simulink model "mc"  (R2025b)
settings: Solver=ode45  StartTime=0.0  StopTime=simlength  MaxStep=1e-4  RelTol=1e-4
values from neighbouring files (symbols this model uses):
  A = [0 1 0;      0 -b/m Bm*h/m;      0 -Bm*h/L -R/L]    [init_moving_coil.m]
  Aled = eye(4) + Ale*Ts    [init_moving_coil.m]
  B = [0 0 1/L]'    [init_moving_coil.m]
  Bled = Ble*Ts    [init_moving_coil.m]
  Bm = 1    [init_moving_coil.m]
  C = [1 0 0; 0 0 1]    [init_moving_coil.m]
  Cle = [1 0 0 0; 0 0 1 0]    [init_moving_coil.m]
  E = [0 -1/m 0]'    [init_moving_coil.m]
  h = 200e-3    (= 0.2)    [init_moving_coil.m]
  Ked = (Ke_hat+[0 0 0 1])/([Ad-eye(3) Bd; C(1,:)*Ad C(1,:)*Bd])    [init_moving_coil.m]
  Lled = place(Aled',Cle',poles_so_led)'    [init_moving_coil.m]
  Tc = 1e-5    (= 1e-05)    [init_moving_coil.m]
  Ts = 1/1e3    (= 0.001)    [init_moving_coil.m]
libraries: ee_lib x1
settings Model: Creator=dabagnara  LastModifiedBy=dbagn
settings SolverCC: AlgebraicLoopSolver=TrustRegion
settings DataIOCC: ReturnWorkspaceOutputs=off
settings DebuggingCC: UnconnectedInputMsg=warning  UnconnectedOutputMsg=warning  UnconnectedLineMsg=warning
settings ModelReferenceCC: EnableRefExpFcnMdlSchedulingChecks=on
settings RTWCC: GPUComputeCapability=3.5

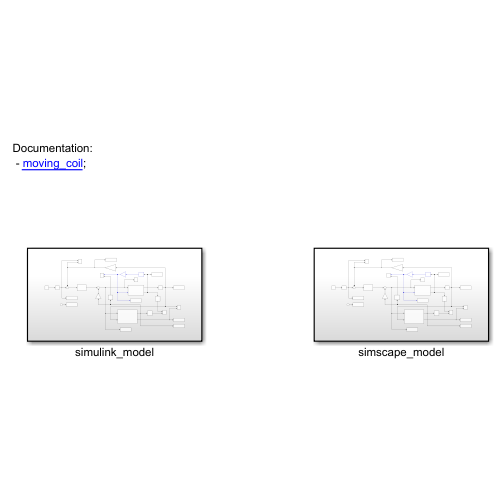
[thumbnail: Simulink's stored preview of the top-level diagram]
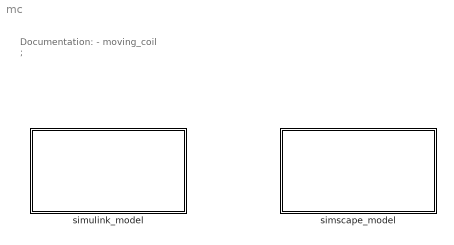
== system mc ==
  note: Documentation:
      | - moving_coil ;
  simscape_model : Subsystem
  simulink_model : Subsystem

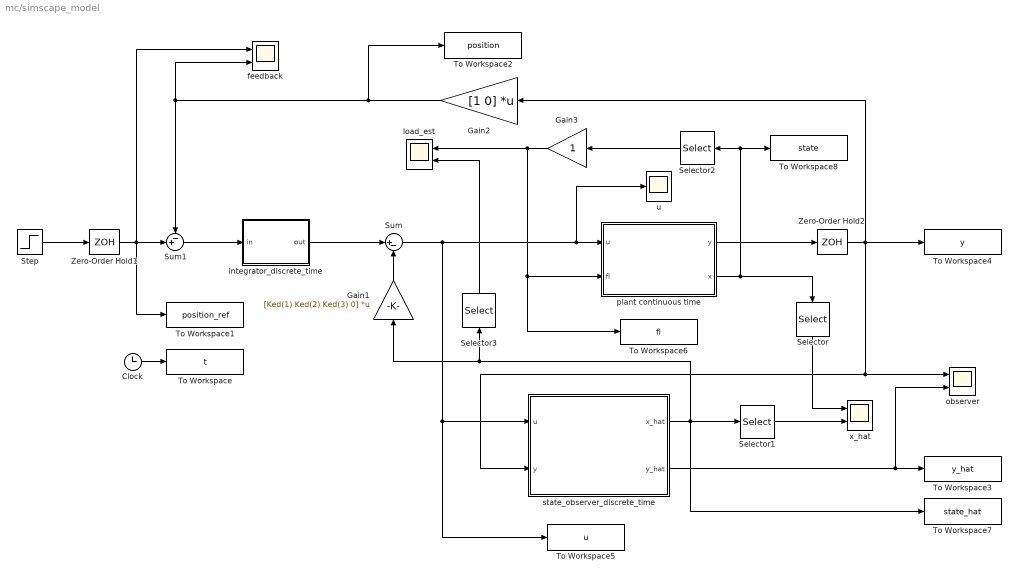
== system mc/simscape_model ==
  Clock : Clock
  Gain1 : Gain  Gain=[Ked(1) Ked(2) Ked(3) 0]  Multiplication=Matrix(K*u)
  Gain2 : Gain  Gain=[1 0]  Multiplication=Matrix(K*u)
  Gain3 : Gain
  Selector : Selector  InputPortWidth=3  IndexOptions=Index vector (dialog)  Indices=2  OutputSizes=1
  Selector1 : Selector  InputPortWidth=4  IndexOptions=Index vector (dialog)  Indices=2  OutputSizes=1
  Selector2 : Selector  InputPortWidth=3  IndexOptions=Index vector (dialog)  Indices=2  OutputSizes=1
  Selector3 : Selector  InputPortWidth=4  IndexOptions=Index vector (dialog)  Indices=4  OutputSizes=1
  Step : Step  Time=0.1  SampleTime=0
  Sum : Sum  Inputs=|+-
  Sum1 : Sum  Inputs=-+|
  To Workspace : ToWorkspace  VariableName=t  SampleTime=Tc
      settings: MaxDataPoints=Nc
  To Workspace1 : ToWorkspace  VariableName=position_ref  SampleTime=Tc
      settings: MaxDataPoints=Nc
  To Workspace2 : ToWorkspace  VariableName=position  SampleTime=Tc
      settings: MaxDataPoints=Nc
  To Workspace3 : ToWorkspace  VariableName=y_hat  SampleTime=Tc
      settings: MaxDataPoints=Nc
  To Workspace4 : ToWorkspace  VariableName=y  SampleTime=Tc
      settings: MaxDataPoints=Nc
  To Workspace5 : ToWorkspace  VariableName=u  SampleTime=Tc
      settings: MaxDataPoints=Nc
  To Workspace6 : ToWorkspace  VariableName=fl  SampleTime=Tc
      settings: MaxDataPoints=Nc
  To Workspace7 : ToWorkspace  VariableName=state_hat  SampleTime=Tc
      settings: MaxDataPoints=Nc
  To Workspace8 : ToWorkspace  VariableName=state  SampleTime=Tc
      settings: MaxDataPoints=Nc
  Zero-Order Hold1 : ZeroOrderHold  SampleTime=Ts
  Zero-Order Hold2 : ZeroOrderHold  SampleTime=Ts
  feedback : Scope  NumInputPorts=2
      settings: ActiveDisplayYMinimum=-0.125  ActiveDisplayYMaximum=1.125
  integrator_discrete_time : Subsystem
  load_est : Scope  NumInputPorts=2
      settings: ActiveDisplayYMinimum=-2.8529  ActiveDisplayYMaximum=14.58894
  observer : Scope  NumInputPorts=2
      settings: ActiveDisplayYMinimum=-11.870884279558481  ActiveDisplayYMaximum=68.425236612925119
  plant continuous time : Subsystem
  state_observer_discrete_time : Subsystem
  u : Scope
      settings: ActiveDisplayYMinimum=-2.39676  ActiveDisplayYMaximum=8.18256  DataLoggingVariableName=ScopeData2
  x_hat : Scope  NumInputPorts=2
      settings: ActiveDisplayYMinimum=-6.8578  ActiveDisplayYMaximum=10.89096  DataLoggingVariableName=ScopeData3
  wires:
  plant continuous time/1(y) -> Zero-Order Hold2/1
  Sum1/1 -> integrator_discrete_time/1(in)
  integrator_discrete_time/1(out) -> Sum/1
  Selector3/1 -> load_est/2
  Selector2/1 -> Gain3/1
  Gain2/1 -> To Workspace2/1, feedback/2, Sum1/1
  Step/1 -> Zero-Order Hold1/1
  Gain1/1 -> Sum/2
  Sum/1 -> state_observer_discrete_time/1(u), To Workspace5/1, plant continuous time/1(u), u/1
  Selector/1 -> x_hat/1
  state_observer_discrete_time/2(y_hat) -> observer/2, To Workspace3/1
  Clock/1 -> To Workspace/1
  Selector1/1 -> x_hat/2
  state_observer_discrete_time/1(x_hat) -> Gain1/1, Selector3/1, To Workspace7/1, Selector1/1
  Zero-Order Hold2/1 -> Gain2/1, To Workspace4/1, observer/1, state_observer_discrete_time/2(y)
  Zero-Order Hold1/1 -> Sum1/2, feedback/1, To Workspace1/1
  Gain3/1 -> load_est/1, To Workspace6/1, plant continuous time/2(fl)
  plant continuous time/2(x) -> Selector/1, Selector2/1, To Workspace8/1

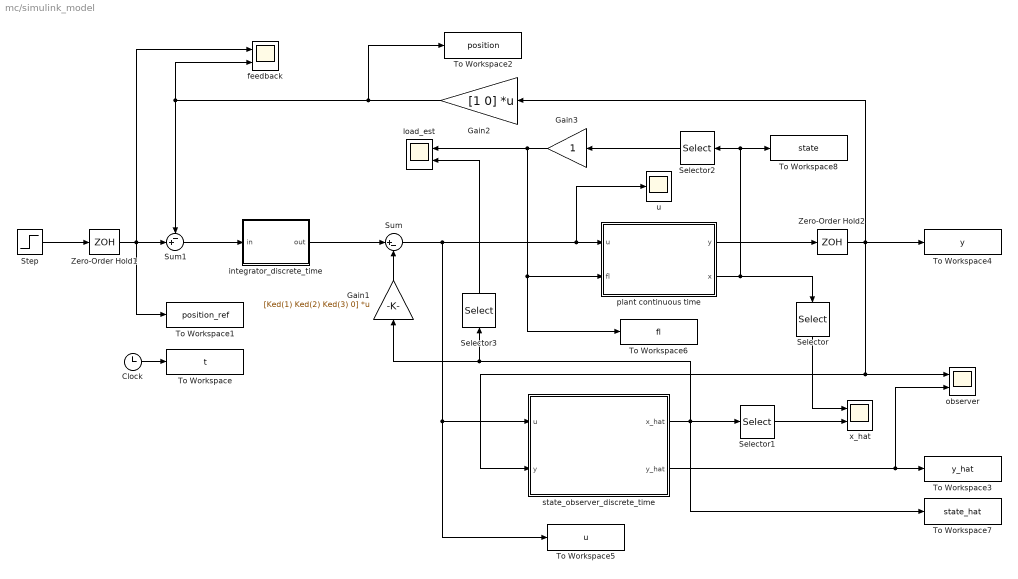
== system mc/simulink_model ==
  Clock : Clock
  Gain1 : Gain  Gain=[Ked(1) Ked(2) Ked(3) 0]  Multiplication=Matrix(K*u)
  Gain2 : Gain  Gain=[1 0]  Multiplication=Matrix(K*u)
  Gain3 : Gain
  Selector : Selector  InputPortWidth=3  IndexOptions=Index vector (dialog)  Indices=2  OutputSizes=1
  Selector1 : Selector  InputPortWidth=4  IndexOptions=Index vector (dialog)  Indices=2  OutputSizes=1
  Selector2 : Selector  InputPortWidth=3  IndexOptions=Index vector (dialog)  Indices=2  OutputSizes=1
  Selector3 : Selector  InputPortWidth=4  IndexOptions=Index vector (dialog)  Indices=4  OutputSizes=1
  Step : Step  Time=0.1  SampleTime=0
  Sum : Sum  Inputs=|+-
  Sum1 : Sum  Inputs=-+|
  To Workspace : ToWorkspace  VariableName=t  SampleTime=Tc
      settings: MaxDataPoints=Nc
  To Workspace1 : ToWorkspace  VariableName=position_ref  SampleTime=Tc
      settings: MaxDataPoints=Nc
  To Workspace2 : ToWorkspace  VariableName=position  SampleTime=Tc
      settings: MaxDataPoints=Nc
  To Workspace3 : ToWorkspace  VariableName=y_hat  SampleTime=Tc
      settings: MaxDataPoints=Nc
  To Workspace4 : ToWorkspace  VariableName=y  SampleTime=Tc
      settings: MaxDataPoints=Nc
  To Workspace5 : ToWorkspace  VariableName=u  SampleTime=Tc
      settings: MaxDataPoints=Nc
  To Workspace6 : ToWorkspace  VariableName=fl  SampleTime=Tc
      settings: MaxDataPoints=Nc
  To Workspace7 : ToWorkspace  VariableName=state_hat  SampleTime=Tc
      settings: MaxDataPoints=Nc
  To Workspace8 : ToWorkspace  VariableName=state  SampleTime=Tc
      settings: MaxDataPoints=Nc
  Zero-Order Hold1 : ZeroOrderHold  SampleTime=Ts
  Zero-Order Hold2 : ZeroOrderHold  SampleTime=Ts
  feedback : Scope  NumInputPorts=2
      settings: ActiveDisplayYMinimum=-0.125  ActiveDisplayYMaximum=1.125
  integrator_discrete_time : Subsystem
  load_est : Scope  NumInputPorts=2
      settings: ActiveDisplayYMinimum=-2.8529  ActiveDisplayYMaximum=14.58894
  observer : Scope  NumInputPorts=2
      settings: ActiveDisplayYMinimum=-11.870884279558481  ActiveDisplayYMaximum=68.425236612925119
  plant continuous time : Subsystem
  state_observer_discrete_time : Subsystem
  u : Scope
      settings: ActiveDisplayYMinimum=-2.39676  ActiveDisplayYMaximum=8.18256  DataLoggingVariableName=ScopeData2
  x_hat : Scope  NumInputPorts=2
      settings: ActiveDisplayYMinimum=-6.8578  ActiveDisplayYMaximum=10.89096  DataLoggingVariableName=ScopeData3
  wires:
  plant continuous time/2(x) -> To Workspace8/1, Selector2/1, Selector/1
  Gain3/1 -> plant continuous time/2(fl), To Workspace6/1, load_est/1
  Zero-Order Hold1/1 -> To Workspace1/1, feedback/1, Sum1/2
  Zero-Order Hold2/1 -> state_observer_discrete_time/2(y), observer/1, To Workspace4/1, Gain2/1
  state_observer_discrete_time/1(x_hat) -> Selector1/1, To Workspace7/1, Selector3/1, Gain1/1
  Selector1/1 -> x_hat/2
  Clock/1 -> To Workspace/1
  state_observer_discrete_time/2(y_hat) -> To Workspace3/1, observer/2
  Selector/1 -> x_hat/1
  Sum/1 -> u/1, plant continuous time/1(u), To Workspace5/1, state_observer_discrete_time/1(u)
  Gain1/1 -> Sum/2
  Step/1 -> Zero-Order Hold1/1
  Gain2/1 -> Sum1/1, feedback/2, To Workspace2/1
  Selector2/1 -> Gain3/1
  Selector3/1 -> load_est/2
  integrator_discrete_time/1(out) -> Sum/1
  Sum1/1 -> integrator_discrete_time/1(in)
  plant continuous time/1(y) -> Zero-Order Hold2/1

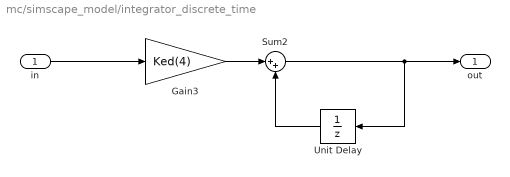
== system mc/simscape_model/integrator_discrete_time ==
  in : Inport
  Gain3 : Gain  Gain=Ked(4)
  Sum2 : Sum  Inputs=|++
  Unit Delay : UnitDelay  SampleTime=Ts  HasFrameUpgradeWarning=on
  out : Outport
  wires:
  Unit Delay/1 -> Sum2/2
  Gain3/1 -> Sum2/1
  in/1 -> Gain3/1
  Sum2/1 -> Unit Delay/1, out/1

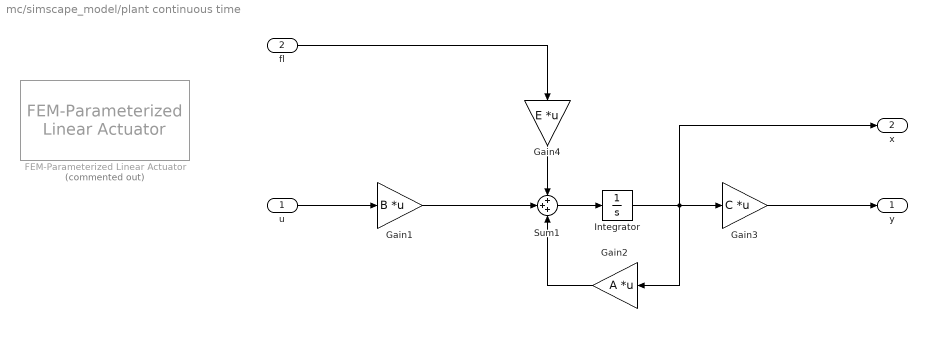
== system mc/simscape_model/plant continuous time ==
  u : Inport
  fl : Inport  Port=2
  FEM-Parameterized Linear Actuator : ee_lib/Electromechanical/Mechatronic Actuators/FEM-Parameterized Linear Actuator  Commented=on  src_type=ee.enum.electromech.femLinearActuator.sourceType.current  iVec=[0, 1] A  xVec=[0, .05, .1, .15, .2] mm  dfluxdiMatrix=L Wb/A  dfluxdxMatrix=Bm*h Wb/m  FluxMatrix=[0, 0, 0, 0, 0; .0085, .0079, .0075, .0071, .0067; .0171, .016, .0151, .0143, .0137; .0254, .0239, .0226, .0215, .0206; .033, .0312, .0297, .0283, .0271; .0396, .0377, .036, .0345, .0331; .0452, .0433, .0415, .0399, .0384; .0495, .0478, .0461, .0446, .0431; .0526, .0512, .0498, .0485, .0472; .0545, .0537, .0528, .0519, .0508; .0554, .0553, .0551, .0548, .0542] Wb  calculate_force_matrix=ee.enum.enable.no  ForceMatrix=[0, 0, 0, 0, 0; -.6, -.5, -.4, -.3, -.3; -2.3, -2, -1.7, -1.4, -1.2; -4.9, -4.3, -3.7, -3.2, -2.7; -8.3, -7.3, -6.4, -5.5, -4.7; -12.2, -10.7, -9.4, -8.2, -7.2; -16.2, -14.4, -12.7, -11.3, -10; -20, -17.9, -15.9, -14.3, -12.9; -23.3, -20.9, -18.8, -17.1, -15.7; -25.7, -23.1, -21.1, -19.4, -18.2; -26.5, -24.1, -22.2, -20.9, -20.1] N  cyclic=ee.enum.isCyclic.unique  interp_method=simscape.enum.interpolation.linear  extrap_method=simscape.enum.extrapolation.linear  R1=14 Ohm  Rm=inf Ohm  lam=1 N*s/m  Mass=0.05 kg  Xmin=0 mm  Xmax=0.2 mm  K_endstop=1e8 N/m  D_endstop=1e4 N*s/m  i_specify=off  i_priority=None  i=0 A  i_nominal_specify=off  i_nominal_value=1  i_nominal_unit=A  F_specify=off  F_priority=None  F=0 N  F_nominal_specify=off  F_nominal_value=1  F_nominal_unit=N  x_specify=off  x_priority=High  x=0 mm  x_nominal_specify=off  x_nominal_value=1  x_nominal_unit=mm  vel_specify=off  vel_priority=High  vel=0 mm/s  vel_nominal_specify=off  vel_nominal_value=1  vel_nominal_unit=mm/s  magnetic_force_specify=off  magnetic_force_priority=None  magnetic_force=0 N  magnetic_force_nominal_specify=off  magnetic_force_nominal_value=1  magnetic_force_nominal_unit=N  alpha=3.93e-3 1/K  Tmeas=25 degC  thermal_mass=100 J/K  T_specify=off  T_priority=High  T=300 K  T_nominal_specify=off  T_nominal_value=1  T_nominal_unit=K
      settings: InternalSimscapePortConfiguration="{\"Bottom\":[],\"Left\":[{\"id\":\"p\",\"label\":\"+\",\"type\":\"foundation.electrical.electrical\"},{\"id\":\"R\",\"label\":\"R\",\"type\":\"foundation.mechanical.translational.translational\"}],\"Right\":[{\"id\":\"n\",\"label\":\"-\",\"type\":\"foundation.electrical.electrical\"},{\"id\":\"C\",\"label\":\"C\",\"type\":\"foundation.mechanical.translational.translational\"}],\"Top\":[]}"
  Gain1 : Gain  Gain=B  Multiplication=Matrix(K*u)
  Gain2 : Gain  Gain=A  Multiplication=Matrix(K*u)
  Gain3 : Gain  Gain=C  Multiplication=Matrix(K*u)
  Gain4 : Gain  Gain=E  Multiplication=Matrix(K*u)
  Integrator : Integrator
  Sum1 : Sum  Inputs=+++
  y : Outport
  x : Outport  Port=2
  wires:
  fl/1 -> Gain4/1
  Gain4/1 -> Sum1/1
  Gain1/1 -> Sum1/2
  Gain2/1 -> Sum1/3
  Gain3/1 -> y/1
  Integrator/1 -> Gain3/1, Gain2/1, x/1
  u/1 -> Gain1/1
  Sum1/1 -> Integrator/1

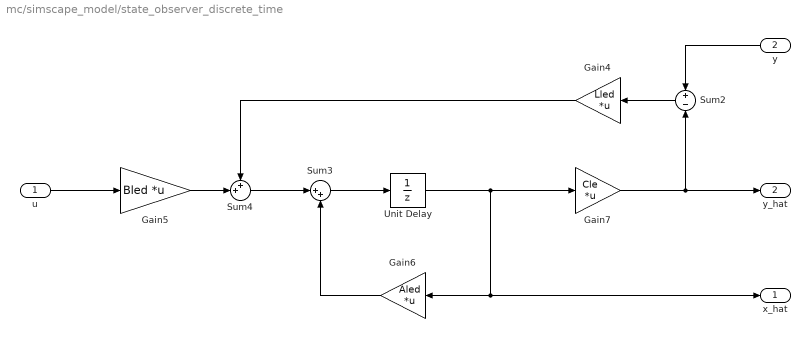
== system mc/simscape_model/state_observer_discrete_time ==
  u : Inport
  y : Inport  Port=2
  Gain4 : Gain  Gain=Lled  Multiplication=Matrix(K*u)
  Gain5 : Gain  Gain=Bled  Multiplication=Matrix(K*u)
  Gain6 : Gain  Gain=Aled  Multiplication=Matrix(K*u)
  Gain7 : Gain  Gain=Cle  Multiplication=Matrix(K*u)
  Sum2 : Sum  Inputs=+-
  Sum3 : Sum  Inputs=|++
  Sum4 : Sum  Inputs=++|
  Unit Delay : UnitDelay  SampleTime=Ts  HasFrameUpgradeWarning=on
  x_hat : Outport
  y_hat : Outport  Port=2
  wires:
  u/1 -> Gain5/1
  Sum4/1 -> Sum3/1
  Gain6/1 -> Sum3/2
  Sum2/1 -> Gain4/1
  Gain5/1 -> Sum4/2
  y/1 -> Sum2/1
  Gain4/1 -> Sum4/1
  Sum3/1 -> Unit Delay/1
  Unit Delay/1 -> x_hat/1, Gain6/1, Gain7/1
  Gain7/1 -> Sum2/2, y_hat/1

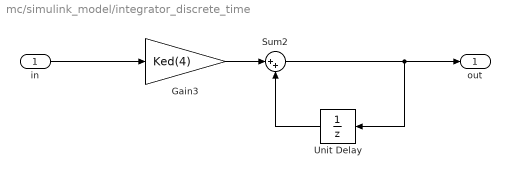
== system mc/simulink_model/integrator_discrete_time ==
  in : Inport
  Gain3 : Gain  Gain=Ked(4)
  Sum2 : Sum  Inputs=|++
  Unit Delay : UnitDelay  SampleTime=Ts  HasFrameUpgradeWarning=on
  out : Outport
  wires:
  Sum2/1 -> out/1, Unit Delay/1
  in/1 -> Gain3/1
  Gain3/1 -> Sum2/1
  Unit Delay/1 -> Sum2/2

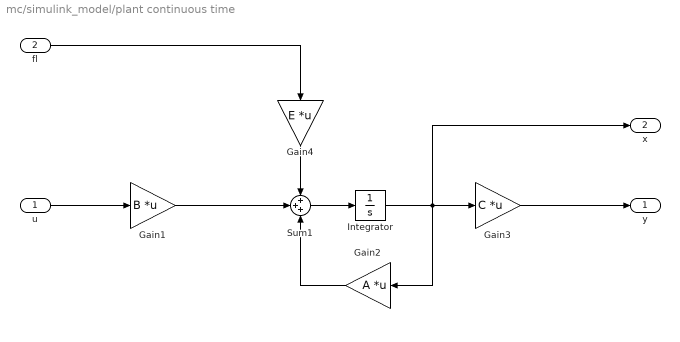
== system mc/simulink_model/plant continuous time ==
  u : Inport
  fl : Inport  Port=2
  Gain1 : Gain  Gain=B  Multiplication=Matrix(K*u)
  Gain2 : Gain  Gain=A  Multiplication=Matrix(K*u)
  Gain3 : Gain  Gain=C  Multiplication=Matrix(K*u)
  Gain4 : Gain  Gain=E  Multiplication=Matrix(K*u)
  Integrator : Integrator
  Sum1 : Sum  Inputs=+++
  y : Outport
  x : Outport  Port=2
  wires:
  Sum1/1 -> Integrator/1
  u/1 -> Gain1/1
  Integrator/1 -> x/1, Gain2/1, Gain3/1
  Gain3/1 -> y/1
  Gain2/1 -> Sum1/3
  Gain1/1 -> Sum1/2
  Gain4/1 -> Sum1/1
  fl/1 -> Gain4/1

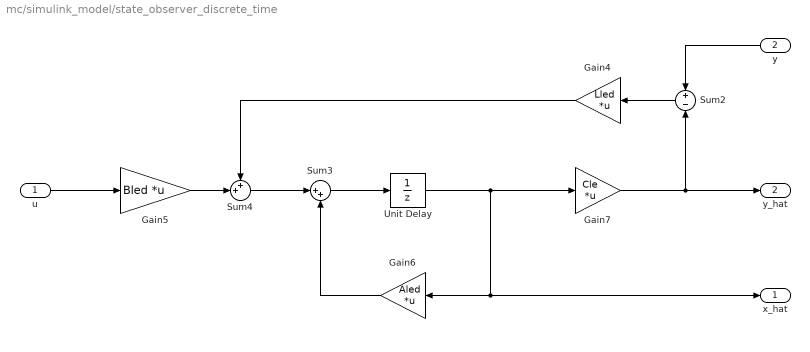
== system mc/simulink_model/state_observer_discrete_time ==
  u : Inport
  y : Inport  Port=2
  Gain4 : Gain  Gain=Lled  Multiplication=Matrix(K*u)
  Gain5 : Gain  Gain=Bled  Multiplication=Matrix(K*u)
  Gain6 : Gain  Gain=Aled  Multiplication=Matrix(K*u)
  Gain7 : Gain  Gain=Cle  Multiplication=Matrix(K*u)
  Sum2 : Sum  Inputs=+-
  Sum3 : Sum  Inputs=|++
  Sum4 : Sum  Inputs=++|
  Unit Delay : UnitDelay  SampleTime=Ts  HasFrameUpgradeWarning=on
  x_hat : Outport
  y_hat : Outport  Port=2
  wires:
  Gain7/1 -> y_hat/1, Sum2/2
  Unit Delay/1 -> Gain7/1, Gain6/1, x_hat/1
  Sum3/1 -> Unit Delay/1
  Gain4/1 -> Sum4/1
  y/1 -> Sum2/1
  Gain5/1 -> Sum4/2
  Sum2/1 -> Gain4/1
  Gain6/1 -> Sum3/2
  Sum4/1 -> Sum3/1
  u/1 -> Gain5/1
